simulink model "PowerModel"  (R2020a)
settings: Solver=VariableStepAuto  StartTime=0.0  StopTime=.5  RelTol=1e-3
libraries: powerlib x60
settings Model: Creator=TommyBoy  LastModifiedBy=TommyBoy

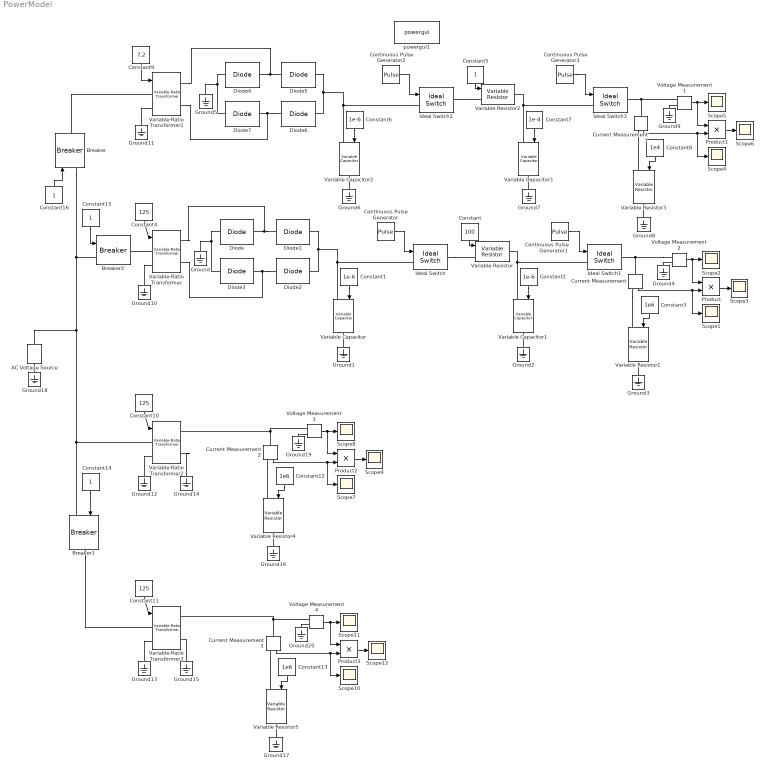
== system PowerModel ==
  AC Voltage Source : powerlib/Electrical Sources/AC Voltage Source  Amplitude=4160  Phase=0  Frequency=60  SampleTime=0  Measurements=None  BusType=PQ  Pref=5e6  Qref=0  Qmin=-inf  Qmax=+inf
  Breaker : powerlib/Elements/Breaker  InitialState=0  SwitchingTimes="[1/60  5/60]"  External=on  BreakerResistance=0.01  SnubberResistance=1e6  SnubberCapacitance=inf  Measurements=None  MoreParameters=on  NoBreakLoop=off
  Breaker1 : powerlib/Elements/Breaker  InitialState=0  SwitchingTimes="[1/60  5/60]"  External=on  BreakerResistance=0.01  SnubberResistance=1e6  SnubberCapacitance=inf  Measurements=None  MoreParameters=on  NoBreakLoop=off
  Breaker2 : powerlib/Elements/Breaker  InitialState=0  SwitchingTimes="[1/60  5/60]"  External=on  BreakerResistance=0.01  SnubberResistance=1e6  SnubberCapacitance=inf  Measurements=None  MoreParameters=on  NoBreakLoop=off
  Constant : Constant  Value=100
  Constant1 : Constant  Value=1e-6
  Constant10 : Constant  Value=125
  Constant11 : Constant  Value=125
  Constant12 : Constant  Value=1e6
  Constant13 : Constant  Value=1e6
  Constant{5,14..16} (4 alike) : Constant
  Constant2 : Constant  Value=1e-6
  Constant3 : Constant  Value=1e6
  Constant4 : Constant  Value=125
  Constant6 : Constant  Value=1e-6
  Constant7 : Constant  Value=1e-4
  Constant8 : Constant  Value=1e4
  Constant9 : Constant  Value=7.2
  Continuous Pulse Generator : DiscretePulseGenerator  PulseType=Time based  Period=50e-3  PulseWidth=50
  Continuous Pulse Generator1 : DiscretePulseGenerator  PulseType=Time based  Period=50e-3  PulseWidth=50  PhaseDelay=25e-3
  Continuous Pulse Generator2 : DiscretePulseGenerator  PulseType=Time based  Period=50e-3  PulseWidth=50
  Continuous Pulse Generator3 : DiscretePulseGenerator  PulseType=Time based  Period=50e-3  PulseWidth=50  PhaseDelay=25e-3
  Current Measurement{,1..3} (4 alike) : powerlib/Measurements/Current Measurement  PhasorSimulation=off  OutputType=Complex  PSBequivalent=0
  Diode{,1..7} (8 alike) : powerlib/Power Electronics/Diode  Ron=0.001  Lon=0  Vf=0.8  IC=0  UseSnubber=0  Rs=500  Cs=250e-9  Measurements=off
  Ground{,1..20} (21 alike) : powerlib/Elements/Ground  LConnTagsString=a
  Ideal Switch{,1..3} (4 alike) : powerlib/Power Electronics/Ideal Switch  Ron=0.001  Lon=0  IC=0  Rs=1e5  Cs=inf  Measurements=off
  Product{,1..3} (4 alike) : Product
  Scope{1..12} (12 alike) : Scope
  Variable Capacitor{,1..3} (4 alike) : powerlib/Elements/Variable Capacitor  methode=Backward Euler  Cabsmin=1e-9  Initialize=off  vC0=0  C0=1e-6  iC0=0
      settings: SourceProductBaseCode=PS
  Variable Resistor : powerlib/Elements/Variable Resistor  Rabsmin=100
      settings: SourceProductBaseCode=PS
  Variable Resistor1 : powerlib/Elements/Variable Resistor  Rabsmin=1e6
      settings: SourceProductBaseCode=PS
  Variable Resistor2 : powerlib/Elements/Variable Resistor  Rabsmin=1
      settings: SourceProductBaseCode=PS
  Variable Resistor3 : powerlib/Elements/Variable Resistor  Rabsmin=1
      settings: SourceProductBaseCode=PS
  Variable Resistor4 : powerlib/Elements/Variable Resistor  Rabsmin=1e6
      settings: SourceProductBaseCode=PS
  Variable Resistor5 : powerlib/Elements/Variable Resistor  Rabsmin=1e6
      settings: SourceProductBaseCode=PS
  Variable-Ratio Transformer{,1..3} (4 alike) : powerlib/Elements/Variable-Ratio Transformer
      settings: SourceProductBaseCode=PS
  Voltage Measurement{1..4} (4 alike) : powerlib/Measurements/Voltage Measurement  PhasorSimulation=off  OutputType=Complex  PSBequivalent=0
  powergui1 : powerlib/powergui  Priority=1  SimulationMode=Discrete  SampleTime=0.001  frequency=60  Iterations=50  frequencyindice=60  Pbase=100e6  ErrMax=1e-4  UnitsV=kV  UnitsW=MW  buscounter=0  FunctionMessages=off  echomessages=off  EnableUseOfTLC=off  CurrentSourceSwitches=off  DisableSnubberDevices=off  DisableRonSwitches=off  DisableVfSwitches=off  DisplayEquations=off  AutomaticDiscreteSolvers=off  SolverType=Tustin/Backward Euler (TBE)  Interpol=off  ExternalGateDelay=off  methode=off  Ts=100  x0status=blocks  SPID=on  SwTol=0  HookPort=off  NonlinearTolerance=1e-4  nMaxIteration=100  ContinueOnMaxIteration=off  RestoreLinks=warning  ResistiveCurrentMeasurement=off  Frange=[0:2:500]  Ylog=off  Xlog=on  ShowGrid=off  save=off  variable=ZData  structure=0  ZoomFFT=off  StartTime=0.0  cycles=1  DisplayStyle=1  fundamental=60  FreqAxis=off  MaxFrequency=1000  frequencyindicesteady=1  RmsSteady=1  display=off
  wires:
  Product/1 -> Scope3/1
  Voltage Measurement2/1 -> Product/1, Scope2/1
  Constant1/1 -> Variable Capacitor/1
  Constant/1 -> Variable Resistor/1
  Constant2/1 -> Variable Capacitor1/1
  Continuous Pulse Generator1/1 -> Ideal Switch1/1
  Constant3/1 -> Variable Resistor1/1
  Continuous Pulse Generator/1 -> Ideal Switch/1
  Current Measurement/1 -> Scope1/1, Product/2
  Constant4/1 -> Variable-Ratio Transformer/1
  Product1/1 -> Scope6/1
  Constant9/1 -> Variable-Ratio Transformer1/1
  Constant8/1 -> Variable Resistor3/1
  Voltage Measurement1/1 -> Product1/1, Scope5/1
  Constant6/1 -> Variable Capacitor2/1
  Constant5/1 -> Variable Resistor2/1
  Constant7/1 -> Variable Capacitor3/1
  Continuous Pulse Generator3/1 -> Ideal Switch3/1
  Current Measurement1/1 -> Scope4/1, Product1/2
  Continuous Pulse Generator2/1 -> Ideal Switch2/1
  Constant10/1 -> Variable-Ratio Transformer2/1
  Constant11/1 -> Variable-Ratio Transformer3/1
  Current Measurement2/1 -> Scope7/1, Product2/2
  Constant12/1 -> Variable Resistor4/1
  Product2/1 -> Scope9/1
  Voltage Measurement3/1 -> Product2/1, Scope8/1
  Current Measurement3/1 -> Scope10/1, Product3/2
  Constant13/1 -> Variable Resistor5/1
  Product3/1 -> Scope12/1
  Voltage Measurement4/1 -> Product3/1, Scope11/1
  Constant14/1 -> Breaker1/1
  Constant15/1 -> Breaker2/1
  Constant16/1 -> Breaker/1
  connections:
  Diode2/RConn1 -- Diode1/RConn1 -- Ideal Switch/LConn1 -- Variable Capacitor/LConn1
  Diode/LConn1 -- Diode3/LConn1 -- Ground/LConn1
  Variable Capacitor1/LConn1 -- Ideal Switch1/LConn1 -- Variable Resistor/RConn1
  Voltage Measurement2/LConn1 -- Ideal Switch1/RConn1 -- Current Measurement/LConn1
  Diode2/LConn1 -- Variable-Ratio Transformer/RConn2 -- Diode3/RConn1
  Diode1/LConn1 -- Diode/RConn1 -- Variable-Ratio Transformer/RConn1
  Current Measurement/RConn1 -- Variable Resistor1/LConn1
  Ground3/LConn1 -- Variable Resistor1/RConn1
  Ground1/LConn1 -- Variable Capacitor/RConn1
  Voltage Measurement2/LConn2 -- Ground4/LConn1
  Ground2/LConn1 -- Variable Capacitor1/RConn1
  Ideal Switch/RConn1 -- Variable Resistor/LConn1
  Diode5/LConn1 -- Diode4/RConn1 -- Variable-Ratio Transformer1/RConn1
  Voltage Measurement1/LConn1 -- Ideal Switch3/RConn1 -- Current Measurement1/LConn1
  Diode6/RConn1 -- Diode5/RConn1 -- Ideal Switch2/LConn1 -- Variable Capacitor2/LConn1
  Variable Capacitor3/LConn1 -- Ideal Switch3/LConn1 -- Variable Resistor2/RConn1
  Diode4/LConn1 -- Diode7/LConn1 -- Ground5/LConn1
  Diode6/LConn1 -- Diode7/RConn1 -- Variable-Ratio Transformer1/RConn2
  Voltage Measurement1/LConn2 -- Ground9/LConn1
  Ground7/LConn1 -- Variable Capacitor3/RConn1
  Ground8/LConn1 -- Variable Resistor3/RConn1
  Current Measurement1/RConn1 -- Variable Resistor3/LConn1
  Ground6/LConn1 -- Variable Capacitor2/RConn1
  Ideal Switch2/RConn1 -- Variable Resistor2/LConn1
  Variable-Ratio Transformer/LConn2 -- Ground10/LConn1
  Variable-Ratio Transformer1/LConn2 -- Ground11/LConn1
  Variable-Ratio Transformer2/LConn2 -- Ground12/LConn1
  Variable-Ratio Transformer3/LConn2 -- Ground13/LConn1
  Variable-Ratio Transformer2/RConn2 -- Ground14/LConn1
  Ground15/LConn1 -- Variable-Ratio Transformer3/RConn2
  Breaker/LConn1 -- Breaker2/LConn1 -- Variable-Ratio Transformer2/LConn1 -- Breaker1/LConn1 -- AC Voltage Source/RConn1
  Breaker1/RConn1 -- Variable-Ratio Transformer3/LConn1
  Breaker2/RConn1 -- Variable-Ratio Transformer/LConn1
  Variable-Ratio Transformer1/LConn1 -- Breaker/RConn1
  Ground18/LConn1 -- AC Voltage Source/LConn1
  Current Measurement2/LConn1 -- Voltage Measurement3/LConn1 -- Variable-Ratio Transformer2/RConn1
  Ground16/LConn1 -- Variable Resistor4/RConn1
  Voltage Measurement3/LConn2 -- Ground19/LConn1
  Current Measurement2/RConn1 -- Variable Resistor4/LConn1
  Voltage Measurement4/LConn1 -- Current Measurement3/LConn1 -- Variable-Ratio Transformer3/RConn1
  Ground17/LConn1 -- Variable Resistor5/RConn1
  Voltage Measurement4/LConn2 -- Ground20/LConn1
  Current Measurement3/RConn1 -- Variable Resistor5/LConn1
